simulink subsystem "RealMovWilly"  (R2021b)
settings: Solver=VariableStepAuto  StartTime=0.0  StopTime=10.0  RelTol=1e-3
settings Model: Creator=yo  LastModifiedBy=yo

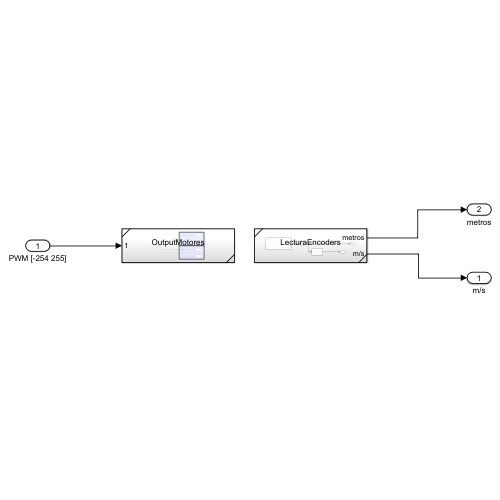
[thumbnail: Simulink's stored preview of the top-level diagram]
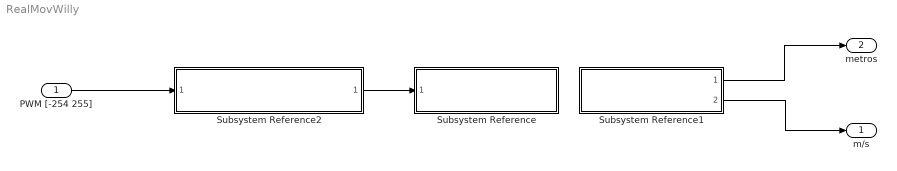
== system RealMovWilly ==
  PWM [-254 255] : Inport
  Subsystem Reference : Subsystem  ReferencedSubsystem=OutputMotores
  Subsystem Reference1 : Subsystem  ReferencedSubsystem=LecturaEncoders
  Subsystem Reference2 : Subsystem  ReferencedSubsystem=CompensadorBateria
  m/s : Outport
  metros : Outport  Port=2
  wires:
  PWM [-254 255]/1 -> Subsystem Reference2/1
  Subsystem Reference1/1 -> metros/1
  Subsystem Reference1/2 -> m/s/1
  Subsystem Reference2/1 -> Subsystem Reference/1
